simulink subsystem "LEDs"  (R2024a)
settings: Solver=VariableStepAuto  StartTime=0.0  StopTime=10.0  RelTol=1e-3
libraries: stm32f4xxblockslib x4
settings Model: Creator=JesseJabezArendse  LastModifiedBy=griff
settings RTWCC: GPUComputeCapability=3.5

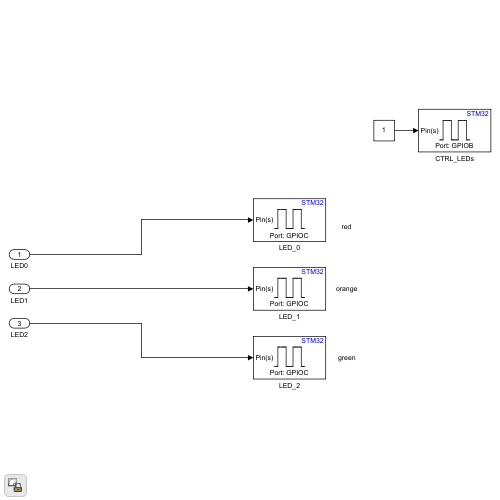
[thumbnail: Simulink's stored preview of the top-level diagram]
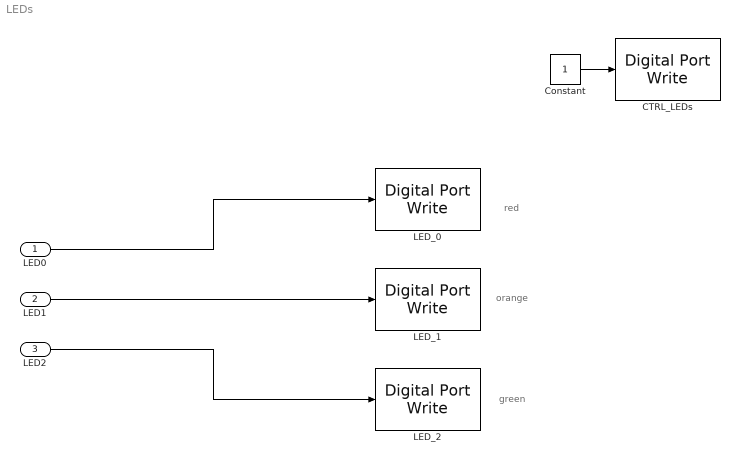
== system LEDs ==
  note: green
  note: orange
  note: red
  LED0 : Inport
  LED1 : Inport  Port=2
  LED2 : Inport  Port=3
  CTRL_LEDs : stm32f4xxblockslib/Digital Port Write  PortName=GPIOB  PinNumber=3  ReadOperation=off  IOAsArray=on  EnableSimPort=off  hoistedMaskSrc=ECSoC/ECSimCodegen/Digital Port Write
      settings: LibrarySourceBlock=stm32l4xxblockslib/Digital Port Write
  Constant : Constant  SampleTime=Inf
  LED_0 : stm32f4xxblockslib/Digital Port Write  PortName=GPIOC  PinNumber=[13]  ReadOperation=off  IOAsArray=on  EnableSimPort=off  hoistedMaskSrc=ECSoC/ECSimCodegen/Digital Port Write
      settings: LibrarySourceBlock=stm32l4xxblockslib/Digital Port Write
  LED_1 : stm32f4xxblockslib/Digital Port Write  PortName=GPIOC  PinNumber=[14]  ReadOperation=off  IOAsArray=on  EnableSimPort=off  hoistedMaskSrc=ECSoC/ECSimCodegen/Digital Port Write
      settings: LibrarySourceBlock=stm32l4xxblockslib/Digital Port Write
  LED_2 : stm32f4xxblockslib/Digital Port Write  PortName=GPIOC  PinNumber=[15]  ReadOperation=off  IOAsArray=on  EnableSimPort=off  hoistedMaskSrc=ECSoC/ECSimCodegen/Digital Port Write
      settings: LibrarySourceBlock=stm32l4xxblockslib/Digital Port Write
  wires:
  Constant/1 -> CTRL_LEDs/1
  LED0/1 -> LED_0/1
  LED1/1 -> LED_1/1
  LED2/1 -> LED_2/1
